simulink model "volt_to_kelv_ramp"  (R2020b)
settings: Solver=VariableStepAuto  StartTime=0.0  StopTime=12.0  FixedStep=1  RelTol=1e-3
libraries: simulink x1
settings Model: Creator=Training  LastModifiedBy=Training

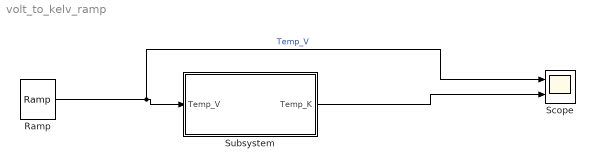
== system volt_to_kelv_ramp ==
  Ramp : simulink/Sources/Ramp  slope=1  start=0  InitialOutput=0
  Scope : Scope  NumInputPorts=2
  Subsystem : Subsystem
  wires:
  Ramp/1 -> Subsystem/1(Temp_V), Scope/1  "Temp_V"
  Subsystem/1(Temp_K) -> Scope/2

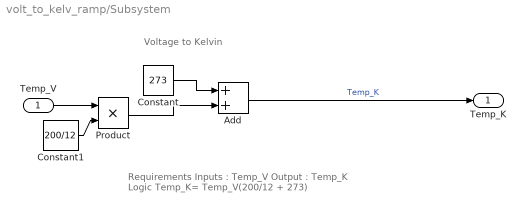
== system volt_to_kelv_ramp/Subsystem ==
  note: Voltage to Kelvin
  note: Requirements
      | Inputs : Temp_V
      | Output : Temp_K
      | Logic
      | Temp_K= Temp_V(200/12 + 273)
  Temp_V : Inport
  Add : Sum
  Constant : Constant  Value=273
  Constant1 : Constant  Value=200/12
  Product : Product
  Temp_K : Outport
  wires:
  Temp_V/1 -> Product/1
  Constant/1 -> Add/1
  Product/1 -> Add/2
  Constant1/1 -> Product/2
  Add/1 -> Temp_K/1  "Temp_K"
